simulink model "chap10_2"  (Simulink 3.00)
settings: Solver=ode45  StartTime=0.0  StopTime=10  RelTol=1e-5

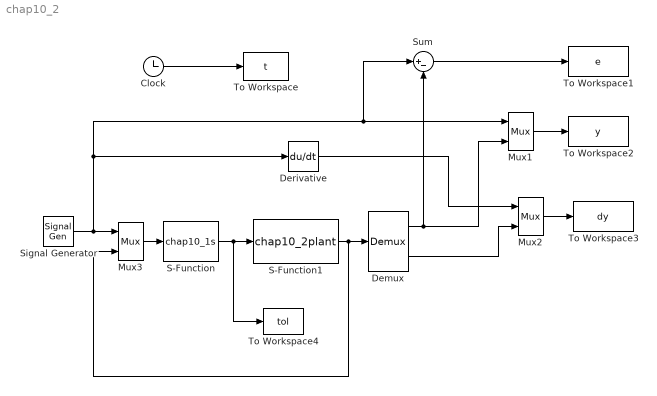
== system chap10_2 ==
  Clock : Clock
      settings: DisplayTime=off  Decimation=10
  Demux : Demux  Outputs=2
  Derivative : Derivative
  Mux1 : Mux  Inputs=2
      settings: DisplayOption=none
  Mux2 : Mux  Inputs=2
      settings: DisplayOption=none
  Mux3 : Mux  Inputs=2
      settings: DisplayOption=none
  S-Function : S-Function  FunctionName=chap10_1s  PortCounts=[]  SFunctionModules=''
  S-Function1 : S-Function  FunctionName=chap10_2plant  PortCounts=[]  SFunctionModules=''
  Signal Generator : SignalGenerator  WaveForm=sine  Amplitude=1  Frequency=1  Units=Hertz
  Sum : Sum  Inputs=|+-  SaturateOnIntegerOverflow=on
  To Workspace : ToWorkspace  VariableName=t  SampleTime=-1  SaveFormat=Matrix
  To Workspace1 : ToWorkspace  VariableName=e  SampleTime=-1  SaveFormat=Matrix
  To Workspace2 : ToWorkspace  VariableName=y  SampleTime=-1  SaveFormat=Matrix
  To Workspace3 : ToWorkspace  VariableName=dy  SampleTime=-1  SaveFormat=Matrix
  To Workspace4 : ToWorkspace  VariableName=tol  SampleTime=-1  SaveFormat=Matrix
  wires:
  Mux1/1 -> To Workspace2/1
  Demux/1 -> Mux1/2, Sum/2
  Sum/1 -> To Workspace1/1
  Mux2/1 -> To Workspace3/1
  Demux/2 -> Mux2/2
  Derivative/1 -> Mux2/1
  S-Function/1 -> S-Function1/1, To Workspace4/1
  S-Function1/1 -> Demux/1, Mux3/2
  Mux3/1 -> S-Function/1
  Signal Generator/1 -> Mux1/1, Sum/1, Derivative/1, Mux3/1
  Clock/1 -> To Workspace/1
